simulink model "pendulum"  (R2024b)
settings: Solver=VariableStepAuto  StartTime=0.0  StopTime=5.0  RelTol=1e-3
undefined symbols (not defined in the file): A, B, F0, x0
settings Model: Creator=Zoran Gaijc  LastModifiedBy=Zoran Gaijc

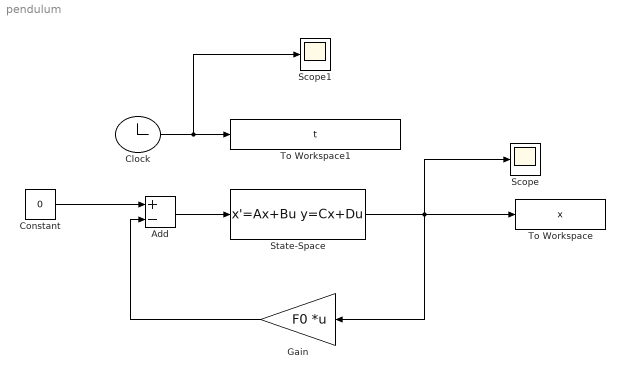
== system pendulum ==
  Add : Sum  Inputs=+-
  Clock : Clock
  Constant : Constant  Value=0
  Gain : Gain  Gain=F0  Multiplication=Matrix(K*u)
  Scope : Scope
  Scope1 : Scope
  State-Space : StateSpace  A=A  B=B  C=eye(4)  D=zeros(4,1)  InitialCondition=x0
  To Workspace : ToWorkspace  VariableName=x  SampleTime=-1
  To Workspace1 : ToWorkspace  VariableName=t  SampleTime=-1
  wires:
  Add/1 -> State-Space/1
  Gain/1 -> Add/2
  State-Space/1 -> Scope/1, To Workspace/1, Gain/1
  Clock/1 -> Scope1/1, To Workspace1/1
  Constant/1 -> Add/1
